simulink model "Duffing"  (R2023a)
settings: Solver=VariableStepAuto  StartTime=0.0  StopTime=10.0  RelTol=1e-3
settings Model: Creator=akb110  LastModifiedBy=akb110

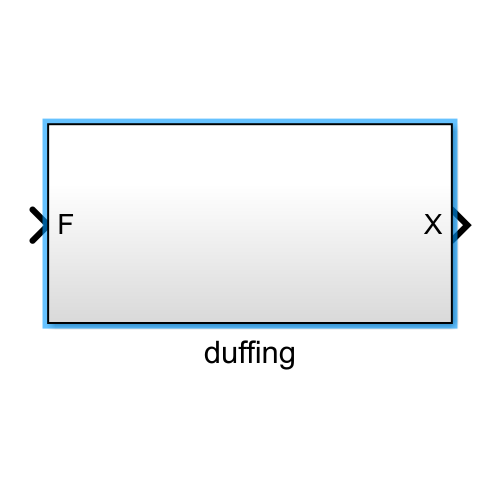
[thumbnail: Simulink's stored preview of the top-level diagram]
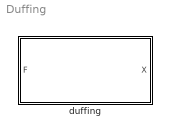
== system Duffing ==
  duffing : Subsystem

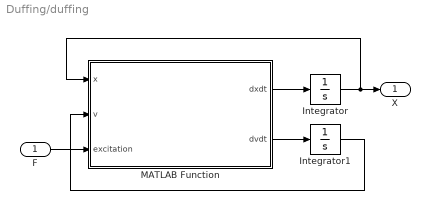
== system Duffing/duffing ==
  F : Inport
  Integrator : Integrator
  Integrator1 : Integrator
  MATLAB Function : MATLAB Function  TreatAsAtomicUnit=on
  X : Outport
  wires:
  Integrator1/1 -> MATLAB Function/2(v)
  MATLAB Function/2(dvdt) -> Integrator1/1
  MATLAB Function/1(dxdt) -> Integrator/1
  F/1 -> MATLAB Function/3(excitation)
  Integrator/1 -> MATLAB Function/1(x), X/1

== matlab function Duffing/duffing/MATLAB Function ==
  data: x input; dxdt output; v input; excitation input; dvdt output
function [dxdt, dvdt] = duffingDerivatives(x, v, excitation)
% Duffing oscillator derivatives
%
% Inputs:
%   x - displacement
%   v - velocity
%   excitation - external excitation signal
%
% Outputs:
%   dx/dt dv/dt

% Define Duffing parameters

% stable duffing
% delta = 0.2;    % damping
% alpha = +1;     % linear stiffness
% beta  = 1;      % nonlinear stiffness

% bi-stable duffing
delta = 0.2;    % damping
alpha = -1;     % linear stiffness
beta  = 1;      % nonlinear stiffness

% bi-stable duffing from Rezaee, Renson: https://doi.org/10.1137/23M1587774
% delta = 0.1;    % damping
% alpha = -4;     % linear stiffness
% beta  = 2;      % nonlinear stiffness


% Duffing equation derivatives
dxdt = v;
dvdt = excitation - delta*v - alpha*x - beta*x^3;

end
